simulink subsystem "execute_command_cgn"  (R2025b)
settings: Solver=VariableStepAuto  StartTime=0.0  StopTime=10.0  RelTol=1e-3
undefined symbols (not defined in the file or in its folder): dt_control
settings Model: Creator=vulcangrip  LastModifiedBy=vulcangrip

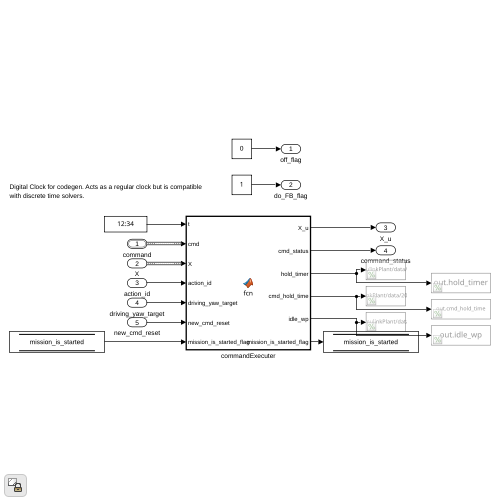
[thumbnail: Simulink's stored preview of the top-level diagram]
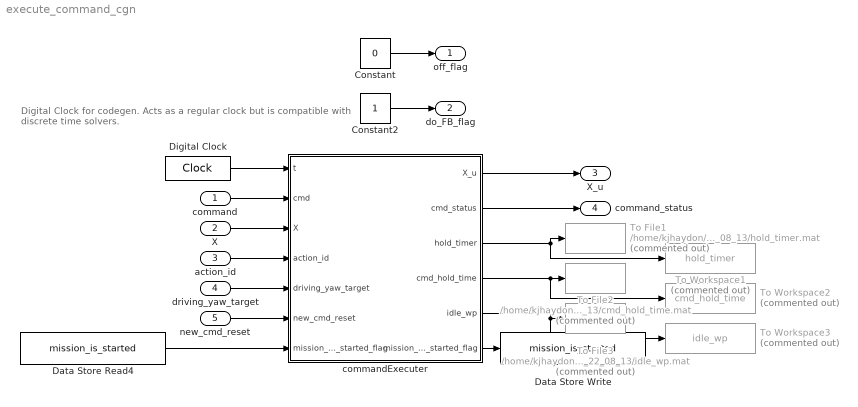
== system execute_command_cgn ==
  note: Digital Clock for codegen. Acts as a regular clock but is compatible
      | with discrete time solvers.
  command : Inport  OutDataTypeStr=Bus: cmd_bus  SampleTime=dt_control
  X : Inport  Port=2  SampleTime=dt_control
  action_id : Inport  Port=3  SampleTime=dt_control
  driving_yaw_target : Inport  Port=4  SampleTime=dt_control
  new_cmd_reset : Inport  Port=5  SampleTime=dt_control
  Constant : Constant  Value=0
  Constant2 : Constant
  Data Store Read4 : DataStoreRead  DataStoreName=mission_is_started  IndexOptions=Index vector (dialog)  Indices=1  OutputSizes=1
  Data Store Write : DataStoreWrite  DataStoreName=mission_is_started  IndexOptions=Index vector (dialog)  Indices=1  OutputSizes=1
  Digital Clock : DigitalClock  SampleTime=dt_control
  To File1 : ToFile  Commented=on  Filename=/home/kjhaydon/Github/Robosub/SimulinkPlant/data/2026_07_06_22_08_13/hold_timer.mat  MatrixName=hold_timer  SaveFormat=Timeseries
  To File2 : ToFile  Commented=on  Filename=/home/kjhaydon/Github/Robosub/SimulinkPlant/data/2026_07_06_22_08_13/cmd_hold_time.mat  MatrixName=cmd_hold_time  SaveFormat=Timeseries
  To File3 : ToFile  Commented=on  Filename=/home/kjhaydon/Github/Robosub/SimulinkPlant/data/2026_07_06_22_08_13/idle_wp.mat  MatrixName=idle_wp  SaveFormat=Timeseries
  To Workspace1 : ToWorkspace  Commented=on  VariableName=hold_timer  SaveFormat=Timeseries  SampleTime=dt_control
  To Workspace2 : ToWorkspace  Commented=on  VariableName=cmd_hold_time  SaveFormat=Timeseries  SampleTime=dt_control
  To Workspace3 : ToWorkspace  Commented=on  VariableName=idle_wp  SaveFormat=Timeseries  SampleTime=dt_control
  commandExecuter : MATLAB Function  TreatAsAtomicUnit=on
  off_flag : Outport
  do_FB_flag : Outport  Port=2
  X_u : Outport  Port=3
  command_status : Outport  Port=4
  wires:
  commandExecuter/4(cmd_hold_time) -> To Workspace2/1, To File2/1
  X/1 -> commandExecuter/3(X)
  commandExecuter/3(hold_timer) -> To Workspace1/1, To File1/1
  Constant/1 -> off_flag/1
  commandExecuter/6(mission_is_started_flag) -> Data Store Write/1
  commandExecuter/5(idle_wp) -> To Workspace3/1, To File3/1
  commandExecuter/1(X_u) -> X_u/1
  commandExecuter/2(cmd_status) -> command_status/1
  command/1 -> commandExecuter/2(cmd)
  Constant2/1 -> do_FB_flag/1
  new_cmd_reset/1 -> commandExecuter/6(new_cmd_reset)
  driving_yaw_target/1 -> commandExecuter/5(driving_yaw_target)
  Data Store Read4/1 -> commandExecuter/7("mission_is_started_flag ")
  action_id/1 -> commandExecuter/4(action_id)
  Digital Clock/1 -> commandExecuter/1(t)

== matlab function execute_command_cgn/commandExecuter ==
  settings: updateMethod=DISCRETE  sampleTime=dt_control
  data: X_u output size=[13 1]; cmd_status output int8 size=[4 1]; hold_timer output; cmd_hold_time output; idle_wp output; t input; cmd input; X input; action_id input; driving_yaw_target input; new_cmd_reset input; mission_is_started_flag input; mission_is_started_flag output
function [X_u, cmd_status, hold_timer, cmd_hold_time, idle_wp, mission_is_started_flag]  = fcn(t, cmd, X, action_id, driving_yaw_target,new_cmd_reset, mission_is_started_flag)

[X_u, cmd_status, hold_timer, cmd_hold_time, idle_wp, mission_is_started_flag] = commandExecuter(t, cmd, X, action_id, driving_yaw_target,new_cmd_reset, mission_is_started_flag);
